simulink model "ekf2"  (R2024b)
settings: Solver=FixedStepAuto  StartTime=0.0  StopTime=10.0  FixedStep=0.005  RelTol=1e-3
undefined symbols (not defined in the file): db
libraries: sharedtransform x1
settings Model: DataDictionary=nextpilot_datadict.sldd  Creator=CETCA  LastModifiedBy=CETCA
settings OptimizationCC: DefaultUnderspecifiedDataType=single

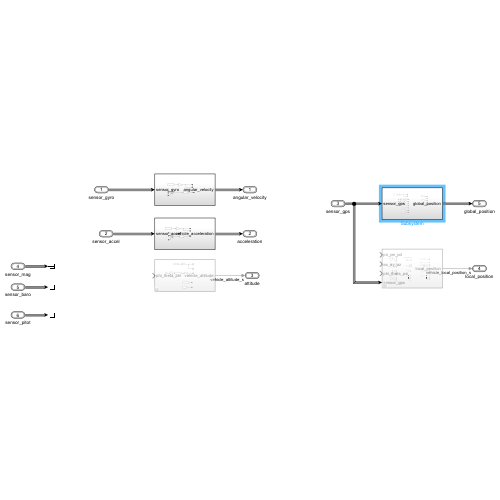
[thumbnail: Simulink's stored preview of the top-level diagram]
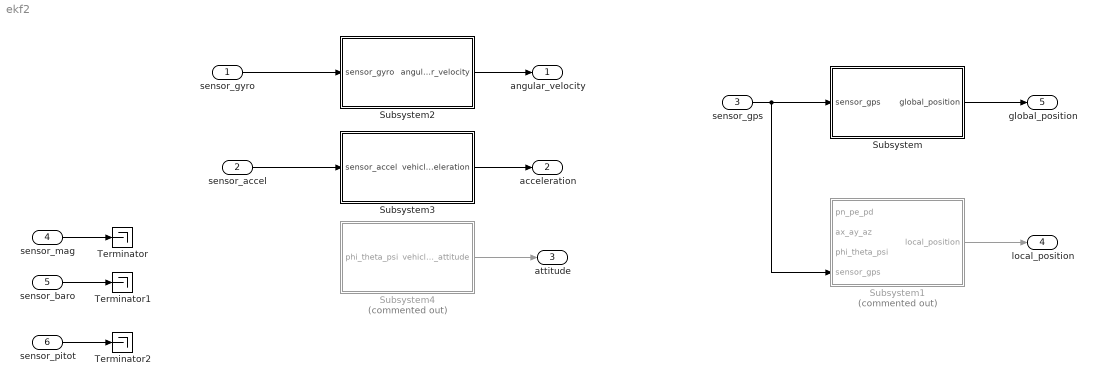
== system ekf2 ==
  sensor_gyro : Inport  OutDataTypeStr=Bus: sensor_gyro_s
  sensor_accel : Inport  Port=2  OutDataTypeStr=Bus: sensor_accel_s
  sensor_gps : Inport  Port=3  OutDataTypeStr=Bus: sensor_gps_s
  sensor_mag : Inport  Port=4  OutDataTypeStr=Bus: sensor_mag_s
  sensor_baro : Inport  Port=5  OutDataTypeStr=Bus: sensor_baro_s
  sensor_pitot : Inport  Port=6  OutDataTypeStr=Bus: differential_pressure_s
  Subsystem : Subsystem
  Subsystem1 : Subsystem  Commented=on
  Subsystem2 : Subsystem
  Subsystem3 : Subsystem
  Subsystem4 : Subsystem  Commented=on
  Terminator : Terminator
  Terminator1 : Terminator
  Terminator2 : Terminator
  angular_velocity : Outport  OutDataTypeStr=Bus: vehicle_angular_velocity_s
  acceleration : Outport  Port=2  OutDataTypeStr=Bus: vehicle_acceleration_s
  attitude : Outport  Port=3  OutDataTypeStr=Bus: vehicle_attitude_s
  local_position : Outport  Port=4  OutDataTypeStr=Bus: vehicle_local_position_s
  global_position : Outport  Port=5  OutDataTypeStr=Bus: vehicle_global_position_s
  wires:
  Subsystem/1(global_position) -> global_position/1
  Subsystem1/1(local_position) -> local_position/1
  Subsystem2/1(angular_velocity) -> angular_velocity/1
  Subsystem3/1(vehicle_acceleration) -> acceleration/1
  Subsystem4/1(vehicle_attitude) -> attitude/1
  sensor_gyro/1 -> Subsystem2/1(sensor_gyro)
  sensor_gps/1 -> Subsystem1/4(sensor_gps), Subsystem/1(sensor_gps)
  sensor_mag/1 -> Terminator/1
  sensor_baro/1 -> Terminator1/1
  sensor_pitot/1 -> Terminator2/1
  sensor_accel/1 -> Subsystem3/1(sensor_accel)

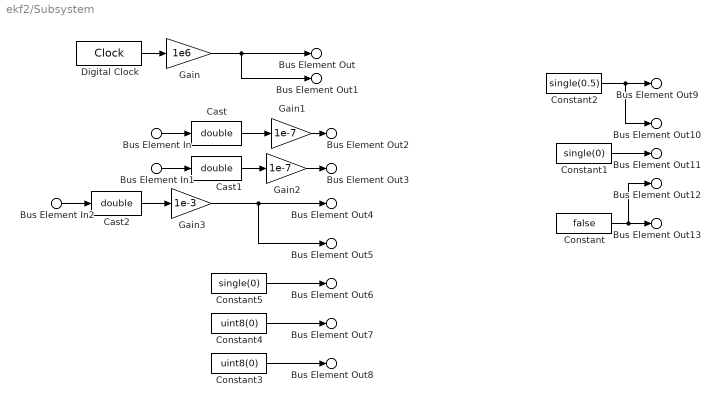
== system ekf2/Subsystem ==
  Bus Element In : Inport  PortName=sensor_gps  Element=lat
  Bus Element In1 : Inport  PortName=sensor_gps  Element=lon
  Bus Element In2 : Inport  PortName=sensor_gps  Element=alt
  Cast : DataTypeConversion  OutDataTypeStr=double  SaturateOnIntegerOverflow=off  RndMeth=Floor
  Cast1 : DataTypeConversion  OutDataTypeStr=double  SaturateOnIntegerOverflow=off  RndMeth=Floor
  Cast2 : DataTypeConversion  OutDataTypeStr=double  SaturateOnIntegerOverflow=off  RndMeth=Floor
  Constant : Constant  Value=false
  Constant1 : Constant  Value=single(0)
  Constant2 : Constant  Value=single(0.5)
  Constant3 : Constant  Value=uint8(0)
  Constant4 : Constant  Value=uint8(0)
  Constant5 : Constant  Value=single(0)
  Digital Clock : DigitalClock
  Gain : Gain  Gain=1e6  OutDataTypeStr=uint64
  Gain1 : Gain  Gain=1e-7  OutDataTypeStr=double
  Gain2 : Gain  Gain=1e-7  OutDataTypeStr=double
  Gain3 : Gain  Gain=1e-3  OutDataTypeStr=single
  Bus Element Out : Outport  PortName=global_position  Element=timestamp
  Bus Element Out1 : Outport  PortName=global_position  Element=timestamp_sample
  Bus Element Out2 : Outport  PortName=global_position  Element=lat
  Bus Element Out3 : Outport  PortName=global_position  Element=lon
  Bus Element Out4 : Outport  PortName=global_position  Element=alt
  Bus Element Out5 : Outport  PortName=global_position  Element=alt_ellipsoid
  Bus Element Out6 : Outport  PortName=global_position  Element=delta_alt
  Bus Element Out7 : Outport  PortName=global_position  Element=lat_lon_reset_counter
  Bus Element Out8 : Outport  PortName=global_position  Element=alt_reset_counter
  Bus Element Out9 : Outport  PortName=global_position  Element=eph
  Bus Element Out10 : Outport  PortName=global_position  Element=epv
  Bus Element Out11 : Outport  PortName=global_position  Element=terrain_alt
  Bus Element Out12 : Outport  PortName=global_position  Element=terrain_alt_valid
  Bus Element Out13 : Outport  PortName=global_position  Element=dead_reckoning
  wires:
  Constant/1 -> Bus Element Out12/1, Bus Element Out13/1
  Constant1/1 -> Bus Element Out11/1
  Constant2/1 -> Bus Element Out10/1, Bus Element Out9/1
  Constant3/1 -> Bus Element Out8/1
  Constant4/1 -> Bus Element Out7/1
  Constant5/1 -> Bus Element Out6/1
  Digital Clock/1 -> Gain/1
  Gain/1 -> Bus Element Out1/1, Bus Element Out/1
  Bus Element In/1 -> Cast/1
  Bus Element In1/1 -> Cast1/1
  Bus Element In2/1 -> Cast2/1
  Gain3/1 -> Bus Element Out5/1, Bus Element Out4/1
  Gain1/1 -> Bus Element Out2/1
  Gain2/1 -> Bus Element Out3/1
  Cast/1 -> Gain1/1
  Cast1/1 -> Gain2/1
  Cast2/1 -> Gain3/1

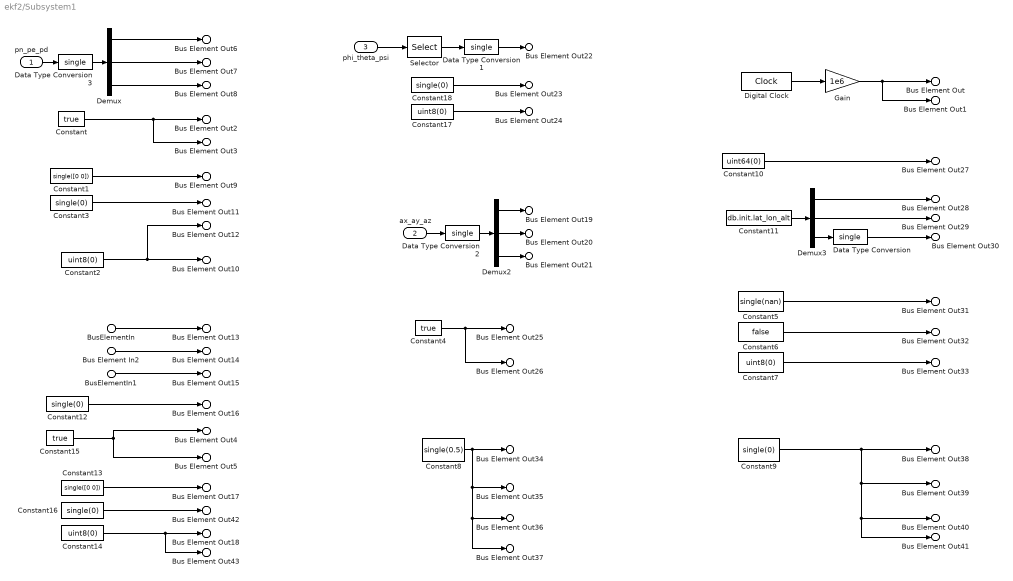
== system ekf2/Subsystem1 ==
  pn_pe_pd : Inport
  ax_ay_az : Inport  Port=2
  phi_theta_psi : Inport  Port=3
  Bus Element In2 : Inport  Port=4  PortName=sensor_gps  Element=vel_e_m_s
  BusElementIn : Inport  Port=4  PortName=sensor_gps  Element=vel_n_m_s
  BusElementIn1 : Inport  Port=4  PortName=sensor_gps  Element=vel_d_m_s
  Constant : Constant  Value=true
  Constant1 : Constant  Value=single([0 0])
  Constant10 : Constant  Value=uint64(0)
  Constant11 : Constant  Value=db.init.lat_lon_alt
  Constant{3,9,12,16,18} (5 alike) : Constant  Value=single(0)
  Constant13 : Constant  Value=single([0 0])
  Constant{2,7,14,17} (4 alike) : Constant  Value=uint8(0)
  Constant15 : Constant  Value=true
  Constant4 : Constant  Value=true
  Constant5 : Constant  Value=single(nan)
  Constant6 : Constant  Value=false
  Constant8 : Constant  Value=single(0.5)
  Data Type Conversion{,1..3} (4 alike) : DataTypeConversion  OutDataTypeStr=single  SaturateOnIntegerOverflow=off  RndMeth=Floor
  Demux : Demux  Outputs=3
  Demux2 : Demux  Outputs=3
  Demux3 : Demux  Outputs=3
  Digital Clock : DigitalClock
  Gain : Gain  Gain=1e6  OutDataTypeStr=uint64
  Selector : Selector  InputPortWidth=3  IndexOptions=Index vector (dialog)  Indices=3  OutputSizes=1
  Bus Element Out : Outport  PortName=local_position  Element=timestamp
  Bus Element Out1 : Outport  PortName=local_position  Element=timestamp_sample
  Bus Element Out2 : Outport  PortName=local_position  Element=xy_valid
  Bus Element Out3 : Outport  PortName=local_position  Element=z_valid
  Bus Element Out4 : Outport  PortName=local_position  Element=v_xy_valid
  Bus Element Out5 : Outport  PortName=local_position  Element=v_z_valid
  Bus Element Out6 : Outport  PortName=local_position  Element=x
  Bus Element Out7 : Outport  PortName=local_position  Element=y
  Bus Element Out8 : Outport  PortName=local_position  Element=z
  Bus Element Out9 : Outport  PortName=local_position  Element=delta_xy
  Bus Element Out10 : Outport  PortName=local_position  Element=xy_reset_counter
  Bus Element Out11 : Outport  PortName=local_position  Element=delta_z
  Bus Element Out12 : Outport  PortName=local_position  Element=z_reset_counter
  Bus Element Out13 : Outport  PortName=local_position  Element=vx
  Bus Element Out14 : Outport  PortName=local_position  Element=vy
  Bus Element Out15 : Outport  PortName=local_position  Element=vz
  Bus Element Out16 : Outport  PortName=local_position  Element=z_deriv
  Bus Element Out17 : Outport  PortName=local_position  Element=delta_vxy
  Bus Element Out18 : Outport  PortName=local_position  Element=vxy_reset_counter
  Bus Element Out42 : Outport  PortName=local_position  Element=delta_vz
  Bus Element Out43 : Outport  PortName=local_position  Element=vz_reset_counter
  Bus Element Out19 : Outport  PortName=local_position  Element=ax
  Bus Element Out20 : Outport  PortName=local_position  Element=ay
  Bus Element Out21 : Outport  PortName=local_position  Element=az
  Bus Element Out22 : Outport  PortName=local_position  Element=heading
  Bus Element Out23 : Outport  PortName=local_position  Element=delta_heading
  Bus Element Out24 : Outport  PortName=local_position  Element=heading_reset_counter
  Bus Element Out25 : Outport  PortName=local_position  Element=xy_global
  Bus Element Out26 : Outport  PortName=local_position  Element=z_global
  Bus Element Out27 : Outport  PortName=local_position  Element=ref_timestamp
  Bus Element Out28 : Outport  PortName=local_position  Element=ref_lat
  Bus Element Out29 : Outport  PortName=local_position  Element=ref_lon
  Bus Element Out30 : Outport  PortName=local_position  Element=ref_alt
  Bus Element Out31 : Outport  PortName=local_position  Element=dist_bottom
  Bus Element Out32 : Outport  PortName=local_position  Element=dist_bottom_valid
  Bus Element Out33 : Outport  PortName=local_position  Element=dist_bottom_sensor_bitfield
  Bus Element Out34 : Outport  PortName=local_position  Element=eph
  Bus Element Out35 : Outport  PortName=local_position  Element=epv
  Bus Element Out36 : Outport  PortName=local_position  Element=evh
  Bus Element Out37 : Outport  PortName=local_position  Element=evv
  Bus Element Out38 : Outport  PortName=local_position  Element=vxy_max
  Bus Element Out39 : Outport  PortName=local_position  Element=vz_max
  Bus Element Out40 : Outport  PortName=local_position  Element=hagl_min
  Bus Element Out41 : Outport  PortName=local_position  Element=hagl_max
  wires:
  Digital Clock/1 -> Gain/1
  Gain/1 -> Bus Element Out1/1, Bus Element Out/1
  Constant/1 -> Bus Element Out3/1, Bus Element Out2/1
  Constant1/1 -> Bus Element Out9/1
  Constant2/1 -> Bus Element Out12/1, Bus Element Out10/1
  Constant3/1 -> Bus Element Out11/1
  Constant4/1 -> Bus Element Out26/1, Bus Element Out25/1
  Constant5/1 -> Bus Element Out31/1
  Constant6/1 -> Bus Element Out32/1
  Constant7/1 -> Bus Element Out33/1
  Constant8/1 -> Bus Element Out37/1, Bus Element Out36/1, Bus Element Out35/1, Bus Element Out34/1
  Constant9/1 -> Bus Element Out39/1, Bus Element Out40/1, Bus Element Out41/1, Bus Element Out38/1
  pn_pe_pd/1 -> Data Type Conversion3/1
  Demux/2 -> Bus Element Out7/1
  Demux/1 -> Bus Element Out6/1
  Demux/3 -> Bus Element Out8/1
  Bus Element In2/1 -> Bus Element Out14/1
  BusElementIn/1 -> Bus Element Out13/1
  BusElementIn1/1 -> Bus Element Out15/1
  Demux2/1 -> Bus Element Out19/1
  Demux2/2 -> Bus Element Out20/1
  Demux2/3 -> Bus Element Out21/1
  ax_ay_az/1 -> Data Type Conversion2/1
  phi_theta_psi/1 -> Selector/1
  Selector/1 -> Data Type Conversion1/1
  Constant10/1 -> Bus Element Out27/1
  Constant11/1 -> Demux3/1
  Demux3/3 -> Data Type Conversion/1
  Demux3/2 -> Bus Element Out29/1
  Demux3/1 -> Bus Element Out28/1
  Data Type Conversion/1 -> Bus Element Out30/1
  Constant12/1 -> Bus Element Out16/1
  Constant13/1 -> Bus Element Out17/1
  Constant14/1 -> Bus Element Out43/1, Bus Element Out18/1
  Constant15/1 -> Bus Element Out5/1, Bus Element Out4/1
  Constant16/1 -> Bus Element Out42/1
  Constant17/1 -> Bus Element Out24/1
  Constant18/1 -> Bus Element Out23/1
  Data Type Conversion1/1 -> Bus Element Out22/1
  Data Type Conversion2/1 -> Demux2/1
  Data Type Conversion3/1 -> Demux/1

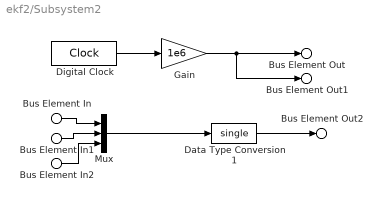
== system ekf2/Subsystem2 ==
  Bus Element In : Inport  PortName=sensor_gyro  Element=x
  Bus Element In1 : Inport  PortName=sensor_gyro  Element=y
  Bus Element In2 : Inport  PortName=sensor_gyro  Element=z
  Data Type Conversion1 : DataTypeConversion  OutDataTypeStr=single  SaturateOnIntegerOverflow=off  RndMeth=Floor
  Digital Clock : DigitalClock
  Gain : Gain  Gain=1e6  OutDataTypeStr=uint64
  Mux : Mux  Inputs=3
  Bus Element Out : Outport  PortName=angular_velocity  Element=timestamp
  Bus Element Out1 : Outport  PortName=angular_velocity  Element=timestamp_sample
  Bus Element Out2 : Outport  PortName=angular_velocity  Element=xyz
  wires:
  Gain/1 -> Bus Element Out1/1, Bus Element Out/1
  Digital Clock/1 -> Gain/1
  Data Type Conversion1/1 -> Bus Element Out2/1
  Mux/1 -> Data Type Conversion1/1
  Bus Element In/1 -> Mux/1
  Bus Element In1/1 -> Mux/2
  Bus Element In2/1 -> Mux/3

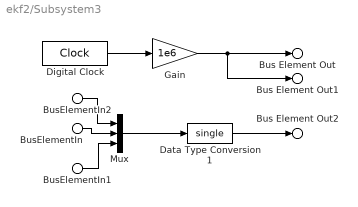
== system ekf2/Subsystem3 ==
  BusElementIn1 : Inport  PortName=sensor_accel  Element=z
  BusElementIn : Inport  PortName=sensor_accel  Element=y
  BusElementIn2 : Inport  PortName=sensor_accel  Element=x
  Data Type Conversion1 : DataTypeConversion  OutDataTypeStr=single  SaturateOnIntegerOverflow=off  RndMeth=Floor
  Digital Clock : DigitalClock
  Gain : Gain  Gain=1e6  OutDataTypeStr=uint64
  Mux : Mux  Inputs=3
  Bus Element Out : Outport  PortName=vehicle_acceleration  Element=timestamp
  Bus Element Out1 : Outport  PortName=vehicle_acceleration  Element=timestamp_sample
  Bus Element Out2 : Outport  PortName=vehicle_acceleration  Element=xyz
  wires:
  Data Type Conversion1/1 -> Bus Element Out2/1
  Digital Clock/1 -> Gain/1
  Gain/1 -> Bus Element Out/1, Bus Element Out1/1
  BusElementIn/1 -> Mux/2
  BusElementIn2/1 -> Mux/1
  BusElementIn1/1 -> Mux/3
  Mux/1 -> Data Type Conversion1/1

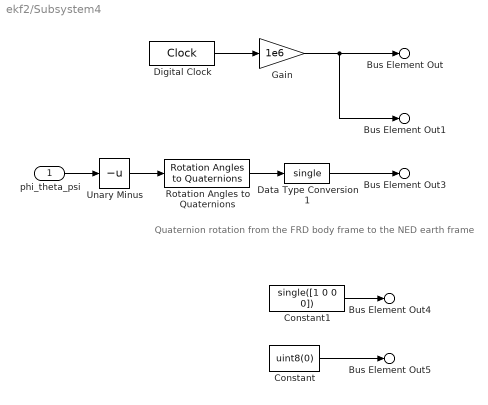
== system ekf2/Subsystem4 ==
  note: Quaternion rotation from the FRD body frame to the NED earth frame
  phi_theta_psi : Inport
  Constant : Constant  Value=uint8(0)
  Constant1 : Constant  Value=single([1 0 0 0])
  Data Type Conversion1 : DataTypeConversion  OutDataTypeStr=single  SaturateOnIntegerOverflow=off  RndMeth=Floor
  Digital Clock : DigitalClock
  Gain : Gain  Gain=1e6  OutDataTypeStr=uint64
  Rotation Angles to Quaternions : sharedtransform/Rotation Angles to Quaternions  rotationOrder=XYZ  aMode=aMode
  Unary Minus : UnaryMinus
  Bus Element Out : Outport  PortName=vehicle_attitude  Element=timestamp
  Bus Element Out1 : Outport  PortName=vehicle_attitude  Element=timestamp_sample
  Bus Element Out3 : Outport  PortName=vehicle_attitude  Element=q
  Bus Element Out4 : Outport  PortName=vehicle_attitude  Element=delta_q_reset
  Bus Element Out5 : Outport  PortName=vehicle_attitude  Element=quat_reset_counter
  wires:
  Gain/1 -> Bus Element Out1/1, Bus Element Out/1
  Digital Clock/1 -> Gain/1
  Constant/1 -> Bus Element Out5/1
  Constant1/1 -> Bus Element Out4/1
  Rotation Angles to Quaternions/1 -> Data Type Conversion1/1
  phi_theta_psi/1 -> Unary Minus/1
  Data Type Conversion1/1 -> Bus Element Out3/1
  Unary Minus/1 -> Rotation Angles to Quaternions/1
